simulink model "ECS_FOS"  (Simulink 8.2)
settings: Solver=ode45  StartTime=0.0  StopTime=18000  RelTol=1e-3
InitFcn:
  | load('loss_coeff_mixing_junction.mat')
  | load('SampleOutput.mat')
  | load('HydProp.mat')
  | load('HydraulicLoad.mat')
  | load('initavload.mat')
  | load('SampleFuelBurn.mat')
values from neighbouring files (symbols this model uses):
  FuelBurn = [0 0 0 0 0 0 0 0 0 0 0 0 ... (18249 elements, 1x18249)]    [Benchmark_data1.mat]
  fueltankdata =     [Benchmark_data1.mat]
undefined symbols (not defined in the file or in its folder): AirProp, F1, F2, HUGHES_TREITLER, magnitude, PN_70147, PumpProp
libraries: PowerFlowLib x46, simulink x4
(part 1 of 5)
settings Model: Creator=mwillms4  LastModifiedBy=mwillms4
settings OptimizationCC: ExpressionDepthLimit=128
settings DebuggingCC: FcnCallInpInsideContextMsg=EnableAllAsWarning  StateNameClashWarn=none

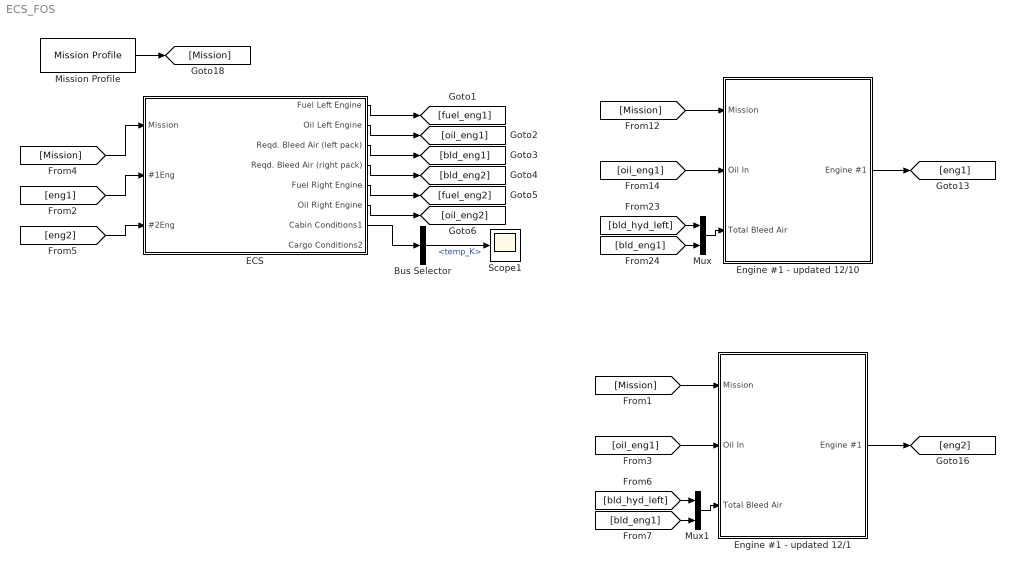
== system ECS_FOS ==
  Bus Selector : BusSelector  OutputSignals=temp_K
  ECS : Subsystem
  Engine #1 - updated 12/1 : Subsystem
  Engine #1 - updated 12/10 : Subsystem
  Mission Profile : PowerFlowLib/Mission Profile/Mission Profile  mssn_check=off  mssn_prof=MSSN  del_P=0  del_T=0  del_rho=0  pres_msl=101.3  temp_msl=15  dens_msl=1.229
  Mux : Mux  Inputs=2
  Mux1 : Mux  Inputs=2
  Scope1 : Scope
      settings: YMin=250  YMax=297.5
  wires:
  Mission Profile/1 -> [Mission]
  [eng1] -> ECS/2(#1Eng)
  [Mission] -> ECS/1(Mission)
  [eng2] -> ECS/3(#2Eng)
  Engine #1 - updated 12/10/1(Engine #1) -> [eng1]
  Engine #1 - updated 12/1/1(Engine #1) -> [eng2]
  [Mission] -> Engine #1 - updated 12/10/1(Mission)
  [oil_eng1] -> Engine #1 - updated 12/10/2(Oil In)
  Mux/1 -> Engine #1 - updated 12/10/3(Total Bleed Air)
  [bld_eng1] -> Mux/2
  [bld_hyd_left] -> Mux/1
  Bus Selector/1 -> Scope1/1  "<temp_K>"
  ECS/1("Fuel Left Engine ") -> [fuel_eng1]
  ECS/2(Oil Left Engine) -> [oil_eng1]
  ECS/3(Reqd. Bleed Air (left pack)) -> [bld_eng1]
  ECS/4(Reqd. Bleed Air (right pack)) -> [bld_eng2]
  ECS/5(Fuel Right Engine) -> [fuel_eng2]
  ECS/6(Oil Right Engine) -> [oil_eng2]
  ECS/7(Cabin Conditions1) -> Bus Selector/1
  [Mission] -> Engine #1 - updated 12/1/1(Mission)
  [oil_eng1] -> Engine #1 - updated 12/1/2(Oil In)
  Mux1/1 -> Engine #1 - updated 12/1/3(Total Bleed Air)
  [bld_eng1] -> Mux1/2
  [bld_hyd_left] -> Mux1/1

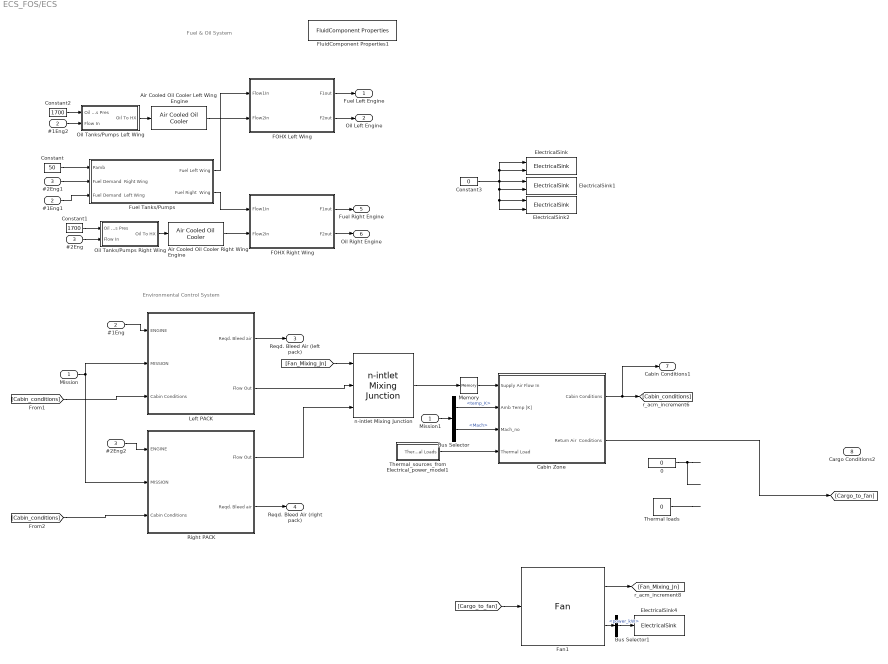
== system ECS_FOS/ECS ==
  note: Fuel & Oil System
  note: Environmental Control System
  Mission : Inport
  #1Eng : Inport  Port=2
  #2Eng : Inport  Port=3
  #1Eng1 : InportShadow  Port=2
  #1Eng2 : InportShadow  Port=2
  #2Eng1 : InportShadow  Port=3
  #2Eng2 : InportShadow  Port=3
  0 : Constant  Value=0
  Air Cooled Oil Cooler Left Wing Engine : PowerFlowLib/Energy & Power Systems/Thermal/Oil/Air Cooled Oil Cooler  fileslct=off  filename=HeatExchangers.mat  filedir=C:\Users\mwillms4\Dropbox\School\Graduate\Research\PowerFlow Summer 2013\PropertyTables\HeatExchangers.mat  refresh=off  hx=HUGHES_TREITLER - PN_70147  bypass_full=1  bypass_none=100  hx_delP=82.74  hx_P=2068  hx_Qdot=24.27  hx_Vdot=0.000505  hx_mass=4.42
  Air Cooled Oil Cooler Right Wing Engine : PowerFlowLib/Energy & Power Systems/Thermal/Oil/Air Cooled Oil Cooler  fileslct=off  filename=HeatExchangers.mat  filedir=C:\Users\mwillms4\Dropbox\School\Graduate\Research\PowerFlow Summer 2013\PropertyTables\HeatExchangers.mat  refresh=off  hx=HUGHES_TREITLER - PN_70147  bypass_full=1  bypass_none=100  hx_delP=82.74  hx_P=2068  hx_Qdot=24.27  hx_Vdot=0.000505  hx_mass=4.42
  Bus Selector : BusSelector  OutputSignals=Flight parameters.temp_K,Flight parameters.Mach
  Bus Selector1 : BusSelector  OutputSignals=power_kW
  Cabin Zone : Subsystem  AncestorBlock=PowerFlowLib/Energy & Power Systems/Thermal/ECS/Cabin Zone  mask(Passenger Cabin){A_fuselage=320, V_cab=130.3, n_pass=176, L_shell=0.003, K_shell=1, L_insulation=0.02, K_insulation=1, L_coating=0.002, K_coating=1, Vdot_sa_pass=0.009438, q_pass=60, RAR=.5, h_outside=1, h_inside=1}
      mask prompts: A_fuselage "Total fuselage area [m^2]"; V_cab "Total cabin volume [m^3]"; n_pass "Total number of passengers [-]"; L_shell "Shell thickness [m]"; K_shell "Shell thermal conductivity [W/m.K]"; L_insulation "Insulation thickness [m]"; K_insulation "Insulation thermal conductivity [W/m.K]"; L_coating "Coating thickness [m]"; K_coating "Coating thermal conductivity [W/m.K]"; Vdot_sa_pass "Required supply air per passenger [m^3/Sec.pass]"; q_pass "Sensible heat release per passenger [W/pass]"; RAR "Recirculation air ratio [-]"; h_outside "Outside convective HT coefficient [W/m^2.K]"; h_inside "Inside convective HT coefficient [W/m^2.K]"
      mask Help:
      | Main assumptions
      | 
      | 1. The thermal loads considered in the current release are: passengers sensible load,
      | wall transmission load, kinetic heating, and electrical/electronic cooling.
      | 2. The actual cabin parameters (fuselage area, air volume, and number of passengers) is split in 2 halves and
      | each half is connected to one of the packs.
      | 3. The cabin model is a single zone model.
      | 4. The wall area is considered constant for the calculation of the overall heat transfer
      | coefficient (i.e. the thickness of the various wall layers is small compared to the
      | shell diameter).
      | 5. The thermal mass of the cabin is considered to be that of the air inside the cabin
      | i.e. neglecting the thermal mass of the structure, furniture, etc.
      | 6. Pressures of: the supply air, recirculation air, exhaust air, and cabin air are
      | considered equal.
      | 7. Temperatures of: exhaust air, and cabin air are considered equal.
      | 8. The management of the equipment thermal load is carried out by the recirculation air rather
      | than the exhaust air. Equipment thermal load management is usually carried out by recirculation
      | air during high cabin pressurization conditions, while exhaust air is used during low cabin
      | pressurization and on-ground conditions.
      | 9. Temperature of the recirculation air is higher than that of the cabin air by the
      | temperature difference due to the equipment theraml load.
      | 10. The themophysical properties (density, and specific heat at constant pressure)
      | of the: recirculation air, exhaust air, and cabin air are based on constant nominal
      | values of air temperature and pressure (T = 298 K, and P = 80 kPa).
      mask Display:
      | image(imread('cabin.png'))
      | port_label('input',1,'{ \bfFlow In}','texmode','on')
      | port_label('input',2,'{ \bfAmbient Temp.}','texmode','on')
      | port_label('input',3,'{ \bfMach #}','texmode','on')
      | port_label('input',4,'{ \bfThermal Loads}','texmode','on')
      | 
      | 
      | port_label('output',1,'{\bfCabin Conditions}','texmode','on')
      | port_label('output',2,'{\bfReturn Air Conditions}','texmode','on')
  Constant : Constant  Value=50
  Constant1 : Constant  Value=1700
  Constant2 : Constant  Value=1700
  Constant3 : Constant  Value=0
  ElectricalSink : PowerFlowLib/Support Functions//Tools/ElectricalSink  Tag=Flow  Description=TwoPhase  load_loc=Empennage  ACDC_load=AC  units=Kilowatts  unq_id=9254
  ElectricalSink1 : PowerFlowLib/Support Functions//Tools/ElectricalSink  Tag=Flow  Description=TwoPhase  load_loc=Cagobay  ACDC_load=AC  units=Kilowatts  unq_id=3572
  ElectricalSink2 : PowerFlowLib/Support Functions//Tools/ElectricalSink  Tag=Flow  Description=TwoPhase  load_loc=Cabin  ACDC_load=AC  units=Kilowatts  unq_id=7814
  ElectricalSink4 : PowerFlowLib/Support Functions//Tools/ElectricalSink  Tag=Flow  Description=TwoPhase  load_loc=Cabin  ACDC_load=DC  units=Kilowatts  unq_id=7783
  FOHX Left Wing : Subsystem  Description=TwoPhase  mask{fld1=JP8, fld2=LubeOil7808, alpha1=80, alpha2=80, N1=10, N2=10, A1_c=.1, A2_c=.1, A1_s=.25, A2_s=.25, P1init=620.5, P2init=620.5}
      mask prompts: fld1 "Fluid 1 Type"; fld2 "Fluid 2 Type"; alpha1 "Fluid 1 HTC [W/m² K]"; alpha2 "Fluid 2 HTC [W/m² K]"; N1 "Flow 1: Number of Channels"; N2 "Flow 2: Number of Channels"; A1_c "Flow 1: Cross-sectional area [m^2]"; A2_c "Flow 2: Cross-sectional area [m^2]"; A1_s "Flow 1: Total surface area [m^2]"; A2_s "Flow 2: Total surface area [m^2]"; P1init "Flow 1 Pressure [kPa]"; P2init "Flow 2 Pressure [kPa]"
      mask init:
      | %load TMSFluidProperties
      | %eval(['SF = FluidProp.SinglePhase.' get_param(gcb,'fld_type1') ';']);
      | %eval(['F = FluidProp.TwoPhase.' get_param(gcb,'fld_type2') ';']);
      | %FluidProp = FluidProp.TwoPhase.R134a; 
      | %{
      | if strcmp(get_param(bdroot,'SimulationStatus'),'initializing') ;
      |     load TwoPhaseProp_Evap
      |     TwoPhaseProp = TwoPhaseProp_Evap;
      |     Evaporator_Init_AFRL;
      | end
      | TMS_SetPhysSigs
      | if strcmp(get_param(gcb,'fld_type1'),'MoistAir')
      |     notair = 0 ; 
      | else
      |     notair = 1 ;
      | end
      | %}
      mask TypeOptions fld1: JP8
      mask TypeOptions fld2: LubeOil7808
      mask Display:
      | port_label('input',1,'Fuel In','TexMode','on') ;
      | port_label('input',2,'Oil In','TexMode','on') ;
      | port_label('output',1,'Fuel Out','TexMode','on') ;
      | port_label('output',2,'Oil Out','TexMode','on') ;
  FOHX Right Wing : Subsystem  Description=TwoPhase  mask{fld1=JP8, fld2=LubeOil7808, alpha1=80, alpha2=80, N1=10, N2=10, A1_c=.1, A2_c=.1, A1_s=.25, A2_s=.25, P1init=620.5, P2init=620.5}
      mask prompts: fld1 "Fluid 1 Type"; fld2 "Fluid 2 Type"; alpha1 "Fluid 1 HTC [W/m² K]"; alpha2 "Fluid 2 HTC [W/m² K]"; N1 "Flow 1: Number of Channels"; N2 "Flow 2: Number of Channels"; A1_c "Flow 1: Cross-sectional area [m^2]"; A2_c "Flow 2: Cross-sectional area [m^2]"; A1_s "Flow 1: Total surface area [m^2]"; A2_s "Flow 2: Total surface area [m^2]"; P1init "Flow 1 Pressure [kPa]"; P2init "Flow 2 Pressure [kPa]"
      mask init: same as ECS_FOS/ECS/FOHX Left Wing
      mask TypeOptions fld1: JP8
      mask TypeOptions fld2: LubeOil7808
      mask Display:
      | port_label('input',1,'Fuel In','TexMode','on') ;
      | port_label('input',2,'Oil In','TexMode','on') ;
      | port_label('output',1,'Fuel Out','TexMode','on') ;
      | port_label('output',2,'Oil Out','TexMode','on') ;
  Fan1 : PowerFlowLib/Energy & Power Systems/Thermal/ECS/Fan  N_fan=1725
  FluidComponent Properties1 : PowerFlowLib/Support Functions//Tools/FluidComponent Properties  fuelprop=FluidProp_JetA3638.mat  oilprop=OilProp.mat  airprop=AirProp.mat  pumpprop=PumpProp.mat  fanprop=Fanmap.mat  compprop=CompProp.mat  heatexprop=HeatExchangers.mat
  Fuel Tanks/Pumps : Subsystem
  Left PACK : Subsystem
  Memory : Memory
  Mission1 : InportShadow
  Oil Tanks/Pumps Left Wing : Subsystem
  Oil Tanks/Pumps Right Wing : Subsystem
  Right PACK : Subsystem
  Thermal loads : Constant  Value=0
  Thermal_sources_from Electrical_power_model1 : Subsystem
  n-intlet Mixing Junction : PowerFlowLib/Energy & Power Systems/Thermal/ECS/n-intlet Mixing Junction  no_inlets=3  d_in_1=0.1  d_in_2=0.1  d_out=0.2
  "Fuel Left Engine " : Outport
  Oil Left Engine : Outport  Port=2
  Reqd. Bleed Air (left pack) : Outport  Port=3
  Reqd. Bleed Air (right pack) : Outport  Port=4
  Fuel Right Engine : Outport  Port=5
  Oil Right Engine : Outport  Port=6
  Cabin Conditions1 : Outport  Port=7
  Cargo Conditions2 : Outport  Port=8
  wires:
  Cabin Zone/2(Return Air  Conditions) -> [Cargo_to_fan]
  Thermal loads/1 -> ?
  Fan1/2 -> Bus Selector1/1
  Fan1/1 -> [Fan_Mixing_Jn]
  [Cargo_to_fan] -> Fan1/1
  Bus Selector1/1 -> ElectricalSink4/1  "<power_kW>"
  Right PACK/1(Flow Out) -> n-intlet Mixing Junction/3
  [Cabin_conditions] -> Left PACK/3(Cabin Conditions)
  [Cabin_conditions] -> Right PACK/3(Cabin Conditions)
  [Fan_Mixing_Jn] -> n-intlet Mixing Junction/1
  Cabin Zone/1(Cabin Conditions) -> [Cabin_conditions], Cabin Conditions1/1
  #2Eng2/1 -> Right PACK/1(ENGINE)
  #1Eng/1 -> Left PACK/1(ENGINE)
  #2Eng/1 -> Oil Tanks/Pumps Right Wing/2(Flow In)
  #1Eng1/1 -> Fuel Tanks/Pumps/3(Fuel Demand  Left Wing)
  #2Eng1/1 -> Fuel Tanks/Pumps/2(Fuel Demand  Right Wing)
  #1Eng2/1 -> Oil Tanks/Pumps Left Wing/2(Flow In)
  Memory/1 -> Cabin Zone/1(Supply Air Flow In)
  Left PACK/2(Flow Out) -> n-intlet Mixing Junction/2
  Bus Selector/2 -> Cabin Zone/3(Mach_no)  "<Mach>"
  Bus Selector/1 -> Cabin Zone/2(Amb Temp [K])  "<temp_K>"
  Mission1/1 -> Bus Selector/1
  n-intlet Mixing Junction/1 -> Memory/1
  Constant3/1 -> ElectricalSink/2, ElectricalSink/1, ElectricalSink1/2, ElectricalSink2/2, ElectricalSink2/1, ElectricalSink1/1
  FOHX Left Wing/2(F2out) -> Oil Left Engine/1
  FOHX Right Wing/2(F2out) -> Oil Right Engine/1
  FOHX Left Wing/1(F1out) -> "Fuel Left Engine "/1
  Fuel Tanks/Pumps/1(Fuel Left Wing) -> FOHX Left Wing/1(Flow1In)
  Constant2/1 -> Oil Tanks/Pumps Left Wing/1(Oil Sys Pres)
  Oil Tanks/Pumps Left Wing/1(Oil To HX) -> Air Cooled Oil Cooler Left Wing Engine/1
  Air Cooled Oil Cooler Left Wing Engine/1 -> FOHX Left Wing/2(Flow2In)
  FOHX Right Wing/1(F1out) -> Fuel Right Engine/1
  Constant1/1 -> Oil Tanks/Pumps Right Wing/1(Oil Sys Pres)
  Oil Tanks/Pumps Right Wing/1(Oil To HX) -> Air Cooled Oil Cooler Right Wing Engine/1
  Fuel Tanks/Pumps/2(Fuel Right  Wing) -> FOHX Right Wing/1(Flow1In)
  Air Cooled Oil Cooler Right Wing Engine/1 -> FOHX Right Wing/2(Flow2In)
  Constant/1 -> Fuel Tanks/Pumps/1(Pamb)
  Right PACK/2(Reqd. Bleed air) -> Reqd. Bleed Air (right pack)/1
  Mission/1 -> Right PACK/2(MISSION), Left PACK/2(MISSION)
  Left PACK/1(Reqd. Bleed air) -> Reqd. Bleed Air (left pack)/1
  ? -> Cargo Conditions2/1
  0/1 -> ?
  Thermal_sources_from Electrical_power_model1/1(Thermal Loads) -> Cabin Zone/4(Thermal Load)

== system ECS_FOS/Engine #1 - updated 12/1 ==
  Mission : Inport
  Oil In : Inport  Port=2
  Total Bleed Air : Inport  Port=3
  Bus Creator : BusCreator  Inputs=3
  Bus Creator1 : BusCreator  Inputs=2
  Bus Creator2 : BusCreator  Inputs=2
  Bus Creator3 : BusCreator
  Bus Selector4 : BusSelector  OutputSignals=Flight parameters.temp_K,Flight parameters.pres_kPa
  Clock : Clock
  Constant1 : Constant  Value=30000
  Constant11 : Constant  Value=90
  Constant2 : Constant  Value=30000
  Gain : Gain
  Gain1 : Gain
  Gain10 : Gain  Gain=6.89475729
  Gain18 : Gain  Gain=2.204622
  Gain2 : Gain
  Gain20 : Gain  Gain=1/ 2.204622
  Gain4 : Gain  Gain=1/ 2.204622
  Gain6 : Gain  Gain=0.5
  Heat Loads : Subsystem
  Isentropic Flow  Equation : Gain  Gain=(3.75)^((1.3-1)/1.3)
  LP CPR : Gain  Gain=3.75
  Lookup Table : Lookup  InputValues=[0:size(FuelBurn,2)-1]  Table=FuelBurn
  Memory : Memory
  Rate Limiter2 : RateLimiter
  Sum of Elements : Sum  Inputs=+
  Engine #1 : Outport
  wires:
  Bus Creator3/1 -> Engine #1/1
  Lookup Table/1 -> Gain6/1
  Clock/1 -> Lookup Table/1
  Bus Selector4/1 -> Isentropic Flow  Equation/1  "<temp_K>"
  Bus Selector4/2 -> LP CPR/1  "<pres_kPa>"
  Mission/1 -> Bus Selector4/1
  Sum of Elements/1 -> Rate Limiter2/1
  Bus Creator2/1 -> Bus Creator3/2  "Fuel"
  Bus Creator1/1 -> Bus Creator3/1  "Spools"
  Bus Creator/1 -> Bus Creator3/3  "Bleed"
  Heat Loads/1(Flow Out) -> Bus Creator3/4  "Oil"
  Oil In/1 -> Memory/1
  Rate Limiter2/1 -> Gain18/1
  Gain18/1 -> Gain1/1  "FlowRateDemand_lb/s"
  Total Bleed Air/1 -> Sum of Elements/1
  Gain/1 -> Bus Creator1/1  "HPSpoolSpeed_rpm"
  Constant1/1 -> Gain/1  "HPSpoolSpeed_rpm"
  Gain2/1 -> Bus Creator1/2  "LPSpoolSpeed_rpm"
  Constant2/1 -> Gain2/1  "LPSpoolSpeed_rpm"
  Gain4/1 -> Bus Creator/1  "BleedAirFlowRate_kgps"
  Gain1/1 -> Gain4/1  "BleedAirFlowRate_lb/s"
  Isentropic Flow  Equation/1 -> Bus Creator/2  "BleedAirTemp_K"
  LP CPR/1 -> Bus Creator/3  "BleedAirPres_kPa"
  Gain20/1 -> Bus Creator2/1  "FuelFlowNeed_kgps"
  Gain6/1 -> Gain20/1  "FuelFlowNeed_lb/s"
  Gain10/1 -> Bus Creator2/2  "FuelLinePres_kPa"
  Constant11/1 -> Gain10/1  "FuelLinePres_psi"
  Memory/1 -> Heat Loads/1(Flow In)

== system ECS_FOS/Engine #1 - updated 12/10 ==
  Mission : Inport
  Oil In : Inport  Port=2
  Total Bleed Air : Inport  Port=3
  Bus Creator : BusCreator  Inputs=3
  Bus Creator1 : BusCreator  Inputs=2
  Bus Creator2 : BusCreator  Inputs=2
  Bus Creator3 : BusCreator
  Bus Selector4 : BusSelector  OutputSignals=Flight parameters.temp_K,Flight parameters.pres_kPa
  Clock : Clock
  Constant1 : Constant  Value=30000
  Constant11 : Constant  Value=90
  Constant2 : Constant  Value=30000
  Gain : Gain
  Gain1 : Gain
  Gain10 : Gain  Gain=6.89475729
  Gain18 : Gain  Gain=2.204622
  Gain2 : Gain
  Gain20 : Gain  Gain=1/ 2.204622
  Gain4 : Gain  Gain=1/ 2.204622
  Gain6 : Gain  Gain=0.5
  Heat Loads : Subsystem
  Isentropic Flow  Equation : Gain  Gain=(3.75)^((1.3-1)/1.3)
  LP CPR : Gain  Gain=3.75
  Lookup Table : Lookup  InputValues=[0:size(FuelBurn,2)-1]  Table=FuelBurn
  Rate Limiter2 : RateLimiter
  Sum of Elements : Sum  Inputs=+
  Engine #1 : Outport
  wires:
  Constant11/1 -> Gain10/1  "FuelLinePres_psi"
  Gain10/1 -> Bus Creator2/2  "FuelLinePres_kPa"
  Gain6/1 -> Gain20/1  "FuelFlowNeed_lb/s"
  Gain20/1 -> Bus Creator2/1  "FuelFlowNeed_kgps"
  LP CPR/1 -> Bus Creator/3  "BleedAirPres_kPa"
  Isentropic Flow  Equation/1 -> Bus Creator/2  "BleedAirTemp_K"
  Gain1/1 -> Gain4/1  "BleedAirFlowRate_lb/s"
  Gain4/1 -> Bus Creator/1  "BleedAirFlowRate_kgps"
  Constant2/1 -> Gain2/1  "LPSpoolSpeed_rpm"
  Gain2/1 -> Bus Creator1/2  "LPSpoolSpeed_rpm"
  Constant1/1 -> Gain/1  "HPSpoolSpeed_rpm"
  Gain/1 -> Bus Creator1/1  "HPSpoolSpeed_rpm"
  Total Bleed Air/1 -> Sum of Elements/1
  Gain18/1 -> Gain1/1  "FlowRateDemand_lb/s"
  Rate Limiter2/1 -> Gain18/1
  Oil In/1 -> Heat Loads/1(Flow In)
  Heat Loads/1(Flow Out) -> Bus Creator3/4  "Oil"
  Bus Creator/1 -> Bus Creator3/3  "Bleed"
  Bus Creator1/1 -> Bus Creator3/1  "Spools"
  Bus Creator2/1 -> Bus Creator3/2  "Fuel"
  Sum of Elements/1 -> Rate Limiter2/1
  Mission/1 -> Bus Selector4/1
  Bus Selector4/2 -> LP CPR/1  "<pres_kPa>"
  Bus Selector4/1 -> Isentropic Flow  Equation/1  "<temp_K>"
  Clock/1 -> Lookup Table/1
  Lookup Table/1 -> Gain6/1
  Bus Creator3/1 -> Engine #1/1

== system ECS_FOS/ECS/Cabin Zone ==
  note: Saturation added to
      | remove division by Zero
  Supply Air Flow In : Inport
  Amb Temp [K] : Inport  Port=2
  Mach_no : Inport  Port=3
  Thermal Load : Inport  Port=4
  Air Properties : Subsystem
  Bias : Bias  Bias=-273.15
  Bus Creator1 : BusCreator
  Bus Creator2 : BusCreator  Inputs=2
  Bus Creator3 : BusCreator  Inputs=3
  Bus Creator4 : BusCreator
  Bus Selector1 : BusSelector  OutputSignals=Cp_ra
  Bus Selector2 : BusSelector  OutputSignals=temp_K,mdot_kgps
  Bus Selector3 : BusSelector  OutputSignals=m_dot_ra
  C to K : Bias  Bias=273.15
  C to K1 : Bias  Bias=273.15
  Cabin Pressurization : Subsystem
  Cabin Temperature : Subsystem
  Cabin_parameters : Subsystem
  Gain : Gain
  Saturation : Saturate  UpperLimit=inf  LowerLimit=eps
  Terminator : Terminator
  calc_recirc_temp_ from_cab_temp : Sum
  data_sink : PowerFlowLib/Support Functions//Tools/data_sink
  m_dot_sa_required1 : Subsystem
  t_sa_term : Product  Inputs=*//
  Cabin Conditions : Outport
  Return Air  Conditions : Outport  Port=2
  wires:
  ? -> Bus Creator4/4  "FlowRates"
  Bus Creator4/1 -> data_sink/1
  Gain/1 -> Bus Creator3/3  "mdot_kgps"
  Bus Creator3/1 -> Return Air  Conditions/1
  Bus Creator2/1 -> Cabin Conditions/1
  Cabin Pressurization/2(Cabin Pres.) -> Bus Creator4/2, Bus Creator3/2, Bus Creator2/1  "pres_kPa"
  Bus Creator1/1 -> Cabin Temperature/4(Air Props.)
  Bus Selector2/2 -> Cabin Pressurization/1(Sup. Air mdot)  "<mdot_kgps>"
  Cabin_parameters/1(Cabin Parameters) -> Cabin Temperature/3(Cabin Param.), Cabin Pressurization/4(Cabin Param.), m_dot_sa_required1/1(Cabin Param.)
  Cabin Pressurization/1(Cabin mdot & mass) -> Cabin Temperature/2(Cabin mdot & mass), [Masses_cabin]
  Air Properties/4(Cabin_AirProp) -> Bus Creator1/1, Cabin Pressurization/3(Cabin Prop.)
  Bus Selector2/1 -> Bias/1  "<temp_K>"
  Air Properties/1(Supply_AirProp) -> Bus Creator1/2, m_dot_sa_required1/2(Sup. Air Prop.)
  Air Properties/2(Recirc_AirProp) -> Bus Creator1/3, Bus Selector1/1
  Air Properties/3(Exhaust_AirProp) -> Bus Creator1/4
  m_dot_sa_required1/1(mdot SA Req.) -> Terminator/1
  Bias/1 -> Cabin Temperature/1(Sup. Air Temp [C])
  C to K/1 -> Bus Creator4/1, Bus Creator2/2  "temp_K"
  Cabin Temperature/1(Cabin Temp. [C]) -> C to K/1, [temp_cabin_C]  "temp_cabin_C"
  [temp_cabin_C] -> Cabin Pressurization/2(Cabin Temp. [C])
  Supply Air Flow In/1 -> Air Properties/1(Supply Air), Bus Selector2/1
  Amb Temp [K]/1 -> Cabin Temperature/5(Amb Temp [K])
  Mach_no/1 -> Cabin Temperature/6(Mach #)
  Thermal Load/1 -> Bus Creator4/3, t_sa_term/1  "Thermal_Load"
  C to K1/1 -> Bus Creator3/1  "temp_K"
  [Masses_cabin] -> Bus Selector3/1
  Bus Selector1/1 -> t_sa_term/2  "<Cp_ra>"
  Bus Selector3/1 -> Gain/1, Saturation/1  "<m_dot_ra>"
  [temp_cabin_C] -> calc_recirc_temp_ from_cab_temp/1
  t_sa_term/1 -> calc_recirc_temp_ from_cab_temp/2
  calc_recirc_temp_ from_cab_temp/1 -> C to K1/1
  Saturation/1 -> t_sa_term/3

== system ECS_FOS/ECS/FOHX Left Wing ==
  Flow1In : Inport
  Flow2In : Inport  Port=2
  Bias : Bias  Bias=-35
  Bias1 : Bias  Bias=-35
  Bus Creator1 : BusCreator  Inputs=6
  Bus Creator2 : BusCreator
  Bus Creator3 : BusCreator
  Bus Selector1 : BusSelector  OutputSignals=h2_out,T2_out
  Bus Selector2 : BusSelector  OutputSignals=mdot_kgps,pres_kPa,temp_K
  Bus Selector3 : BusSelector  OutputSignals=mdot2_in
  Bus Selector5 : BusSelector  OutputSignals=mdot_kgps,temp_K,pres_kPa
  Bus Selector7 : BusSelector  OutputSignals=h1_out,T1_out
  Bus Selector9 : BusSelector  OutputSignals=mdot1_in
  Gain{,1..13} (14 alike) : Gain
  HX_Calcs : Subsystem
  F1out : Outport
  F2out : Outport  Port=2
  wires:
  Bus Selector7/2 -> Gain9/1  "<T1_out>"
  Bus Selector7/1 -> Gain10/1  "<h1_out>"
  Bus Selector9/1 -> Gain12/1  "<mdot1_in>"
  [Outputs] -> Bus Selector7/1
  Gain9/1 -> Bus Creator3/4  "temp_K"
  Gain10/1 -> Bus Creator3/3  "h_kJ/kg"
  Gain12/1 -> Bus Creator3/2  "mdot_kgps"
  Bus Creator3/1 -> F1out/1
  Bus Creator2/1 -> F2out/1
  Bus Selector5/1 -> Gain4/1  "<mdot_kgps>"
  Bus Selector5/2 -> Gain6/1  "<temp_K>"
  Flow2In/1 -> Bus Selector5/1
  Bus Selector2/3 -> Gain2/1  "<temp_K>"
  Bus Selector2/2 -> Gain1/1  "<pres_kPa>"
  Bus Selector2/1 -> Gain/1  "<mdot_kgps>"
  Bus Creator1/1 -> HX_Calcs/1(Inputs), Bus Selector9/1, Bus Selector3/1
  Flow1In/1 -> Bus Selector2/1
  HX_Calcs/1(Out) -> [Outputs]
  Gain6/1 -> Bus Creator1/5  "T2_in"
  Gain4/1 -> Bus Creator1/4  "mdot2_in"
  Gain2/1 -> Bus Creator1/3  "T1_in"
  Gain1/1 -> Bus Creator1/2, Bias1/1  "P1_in"
  Gain/1 -> Bus Creator1/1  "mdot1_in"
  Bus Selector5/3 -> Gain3/1  "<pres_kPa>"
  Gain3/1 -> Bus Creator1/6, Gain13/1  "P2_in"
  Bus Selector1/2 -> Gain7/1  "<T2_out>"
  Bus Selector1/1 -> Gain5/1  "<h2_out>"
  [Outputs] -> Bus Selector1/1
  Gain7/1 -> Bus Creator2/4  "temp_K"
  Gain5/1 -> Bus Creator2/3  "h_kJ/kg"
  Bus Selector3/1 -> Gain8/1  "<mdot2_in>"
  Gain8/1 -> Bus Creator2/2  "mdot_kgps"
  Gain11/1 -> Bus Creator3/1  "pres_kPa"
  Gain13/1 -> Bias/1  "pres_kPa"
  Bias/1 -> Bus Creator2/1  "pres_kPa"
  Bias1/1 -> Gain11/1

== system ECS_FOS/ECS/FOHX Right Wing ==
  Flow1In : Inport
  Flow2In : Inport  Port=2
  Bias : Bias  Bias=-35
  Bias1 : Bias  Bias=-35
  Bus Creator1 : BusCreator  Inputs=6
  Bus Creator2 : BusCreator
  Bus Creator3 : BusCreator
  Bus Selector1 : BusSelector  OutputSignals=h2_out,T2_out
  Bus Selector2 : BusSelector  OutputSignals=mdot_kgps,pres_kPa,temp_K
  Bus Selector3 : BusSelector  OutputSignals=mdot2_in
  Bus Selector5 : BusSelector  OutputSignals=mdot_kgps,temp_K,pres_kPa
  Bus Selector7 : BusSelector  OutputSignals=h1_out,T1_out
  Bus Selector9 : BusSelector  OutputSignals=mdot1_in
  Gain{,1..13} (14 alike) : Gain
  HX_Calcs : Subsystem
  F1out : Outport
  F2out : Outport  Port=2
  wires:
  Bias1/1 -> Gain11/1
  Bias/1 -> Bus Creator2/1  "pres_kPa"
  Gain13/1 -> Bias/1  "pres_kPa"
  Gain11/1 -> Bus Creator3/1  "pres_kPa"
  Gain8/1 -> Bus Creator2/2  "mdot_kgps"
  Bus Selector3/1 -> Gain8/1  "<mdot2_in>"
  Gain5/1 -> Bus Creator2/3  "h_kJ/kg"
  Gain7/1 -> Bus Creator2/4  "temp_K"
  [Outputs] -> Bus Selector1/1
  Bus Selector1/1 -> Gain5/1  "<h2_out>"
  Bus Selector1/2 -> Gain7/1  "<T2_out>"
  Gain3/1 -> Gain13/1, Bus Creator1/6  "P2_in"
  Bus Selector5/3 -> Gain3/1  "<pres_kPa>"
  Gain/1 -> Bus Creator1/1  "mdot1_in"
  Gain1/1 -> Bias1/1, Bus Creator1/2  "P1_in"
  Gain2/1 -> Bus Creator1/3  "T1_in"
  Gain4/1 -> Bus Creator1/4  "mdot2_in"
  Gain6/1 -> Bus Creator1/5  "T2_in"
  HX_Calcs/1(Out) -> [Outputs]
  Flow1In/1 -> Bus Selector2/1
  Bus Creator1/1 -> Bus Selector3/1, Bus Selector9/1, HX_Calcs/1(Inputs)
  Bus Selector2/1 -> Gain/1  "<mdot_kgps>"
  Bus Selector2/2 -> Gain1/1  "<pres_kPa>"
  Bus Selector2/3 -> Gain2/1  "<temp_K>"
  Flow2In/1 -> Bus Selector5/1
  Bus Selector5/2 -> Gain6/1  "<temp_K>"
  Bus Selector5/1 -> Gain4/1  "<mdot_kgps>"
  Bus Creator2/1 -> F2out/1
  Bus Creator3/1 -> F1out/1
  Gain12/1 -> Bus Creator3/2  "mdot_kgps"
  Gain10/1 -> Bus Creator3/3  "h_kJ/kg"
  Gain9/1 -> Bus Creator3/4  "temp_K"
  [Outputs] -> Bus Selector7/1
  Bus Selector9/1 -> Gain12/1  "<mdot1_in>"
  Bus Selector7/1 -> Gain10/1  "<h1_out>"
  Bus Selector7/2 -> Gain9/1  "<T1_out>"
